simulink model "delay"  (Simulink 6.5)
settings: Solver=ode4  StartTime=0.0  StopTime=10.0  FixedStep=0.1  RelTol=1e-3
settings Model: Creator=vjoel  LastModifiedBy=vjoel

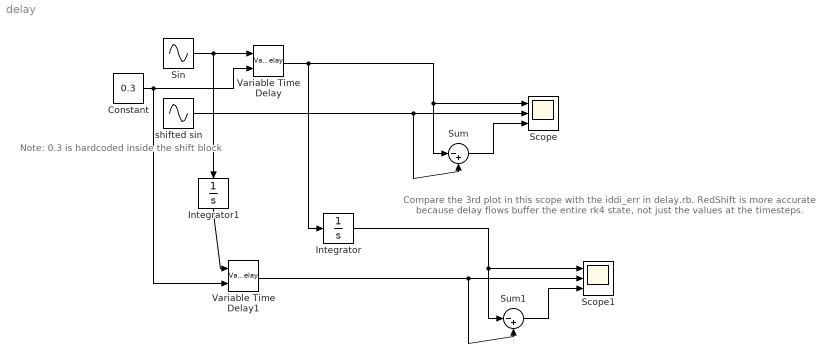
== system delay ==
  note: Note: 0.3 is
      | hardcoded
      | inside the
      | shift block
  note: Compare the 3rd plot in this scope
      | with the iddi_err in delay.rb.
      | RedShift is more accurate
      | because delay flows buffer
      | the entire rk4 state, not
      | just the values at the timesteps.
  Constant : Constant  Value=0.3  OutDataType=sfix(16)  ConRadixGroup=Use specified scaling  OutScaling=2^0  SampleTime=inf  FramePeriod=inf
  Integrator : Integrator
  Integrator1 : Integrator  Orientation=down
  Scope : Scope  NumInputPorts=3
      settings: YMin=-5~-5~-5  YMax=5~5~5
  Scope1 : Scope  NumInputPorts=3
      settings: YMin=-5~-5~-5  YMax=5~5~5
  Sin : Sin  Frequency=pi/2  SampleTime=0
  Sum : Sum  Inputs=|-+
  Sum1 : Sum  Inputs=|-+
  Variable Time Delay : VariableTransportDelay  MaximumDelay=10
  Variable Time Delay1 : VariableTransportDelay  MaximumDelay=10
  shifted sin : Sin  Frequency=pi/2  Phase=-0.3 * pi/2  SampleTime=0
  wires:
  Sin/1 -> Variable Time Delay/1, Integrator1/1
  Variable Time Delay/1 -> Scope/1, Sum/1, Integrator/1
  shifted sin/1 -> Scope/2, Sum/2
  Sum/1 -> Scope/3
  Constant/1 -> Variable Time Delay/2, Variable Time Delay1/2
  Integrator/1 -> Scope1/1, Sum1/1
  Variable Time Delay1/1 -> Scope1/2, Sum1/2
  Sum1/1 -> Scope1/3
  Integrator1/1 -> Variable Time Delay1/1
